simulink model "pe_pmsm_drive_project"  (R2018b)
settings: Solver=FixedStepAuto  StartTime=0.0  StopTime=0.5  FixedStep=2e-7  MaxStep=2.0E-6  RelTol=1e-6  AbsTol=1e-3  EnableMultiTasking=on
PreLoadFcn:
  | % Control parameters
  | Ts = 2e-6;   % Fundamental sample time
  | fsw = 2e3;   % Switching frequency (Hz)
  | fc = fsw*10; % Control loop frequency (Hz)
  | Tsc = 1/fc;  % Control loop sample time
  | 
  | % PMSM parameters
  | PM = 0.03; % Permanent magnet flux linkage
  | Ld = 2e-4;  % d-axis inductance
  | Lq = 2e-4;  % q-axis inductance
  | L0 = 2e-4;  % 0-axis inductance
  | Rs = 0.013; % Stator resistance
  | N = 6; % Number of pole pairs
  | J = 0.2; % Moment of inertia
  | 
  | % Operating and derived limits
  | Imax = 100;  % Max stator current (peak value)
  | Tmax = 1.5*N*PM*Imax; % Max lectromagnetic torque
  | fnom = 100;  % Nominal frequency (Hz)
  | rpm_nom = 60*fnom/N;      % Nominal rotor speed (rpm)
  | omegam_nom = 2*pi*fnom/N; % Nominal mechanical rotor speed
  | Pmax = omegam_nom*Tmax;     % Maximum power
undefined symbols (not defined in the file): faero, gcbh, pe_sli_rtmsupport, speed, wheelrad
libraries: nesl_utility x12, pe_lib x10, fl_lib x8, peTransforms x2, pePmsmCurrentController x1, simulink x1, peVelocityController x1, pePwmGeneratorTwoLevel x1, discretizing x1
(part 2 of 2)

== system pe_pmsm_drive_project/PMSM controller/PMSM Field-Oriented Control/Outer loop control/Tq Selector ==
  Reference : Inport
  TqRefUnsat : Inport  Port=2
  Constant : Constant  Value=CtrlMode  SampleTime=Tsc
  Switch : Switch  Criteria=u2 > Threshold  Threshold=1.5
  TqRef : Outport
  wires:
  Switch/1 -> TqRef/1
  Constant/1 -> Switch/2
  TqRefUnsat/1 -> Switch/3
  Reference/1 -> Switch/1

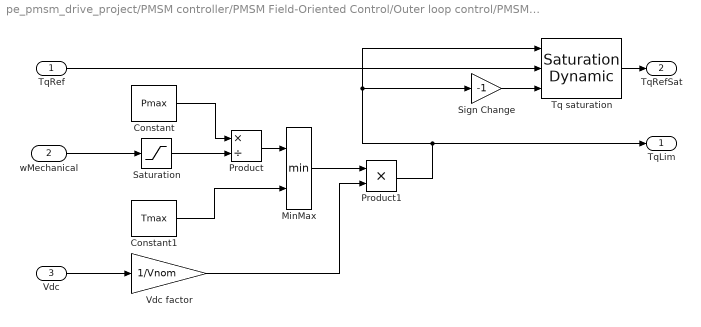
== system pe_pmsm_drive_project/PMSM controller/PMSM Field-Oriented Control/Outer loop control/PMSM Current Reference Generator/Torque limiter ==
  TqRef : Inport
  wMechanical : Inport  Port=2
  Vdc : Inport  Port=3
  Constant : Constant  Value=Pmax  SampleTime=Ts
  Constant1 : Constant  Value=Tmax  SampleTime=Ts
  MinMax : MinMax  Inputs=2
  Product : Product  Inputs=*/
  Product1 : Product
  Saturation : Saturate  UpperLimit=inf  LowerLimit=Pmax/Tmax
  Sign Change : Gain  Gain=-1
  Tq saturation : simulink/Discontinuities/Saturation Dynamic  OutMin=[]  OutMax=[]  OutDataTypeStr=Inherit: Same as second input  OutDataType=fixdt(1, 16)  OutScaling=2^-10  DoSatur=off
  Vdc factor : Gain  Gain=1/Vnom
  TqLim : Outport
  TqRefSat : Outport  Port=2
  wires:
  Tq saturation/1 -> TqRefSat/1
  Vdc/1 -> Vdc factor/1
  Constant1/1 -> MinMax/2
  wMechanical/1 -> Saturation/1
  Product/1 -> MinMax/1
  Constant/1 -> Product/1
  Saturation/1 -> Product/2
  Sign Change/1 -> Tq saturation/3
  MinMax/1 -> Product1/1
  Vdc factor/1 -> Product1/2
  TqRef/1 -> Tq saturation/2
  Product1/1 -> Sign Change/1, Tq saturation/1, TqLim/1
